simulink model "Practica_3_slm"  (R2022a)
settings: Solver=VariableStepAuto  StartTime=0.0  StopTime=10.0  RelTol=1e-3
values from neighbouring files (symbols this model uses):
  b1 = 1000    [Practica_3_codigo_sml.m]    (also in Practica_3_fx.m)
  f = 0    [Practica_3_codigo_sml.m]    (also in Practica_3_fx.m)
  k1 = 16182    [Practica_3_codigo_sml.m]    (also in Practica_3_fx.m)
  k2 = 19000    [Practica_3_codigo_sml.m]    (also in Practica_3_fx.m)
  m1 = 290    [Practica_3_codigo_sml.m]    (also in Practica_3_fx.m)
  m2 = 59    [Practica_3_codigo_sml.m]    (also in Practica_3_fx.m)
libraries: fl_lib x11, nesl_utility x4
settings Model: Creator=Peri_XP  LastModifiedBy=Peri_XP

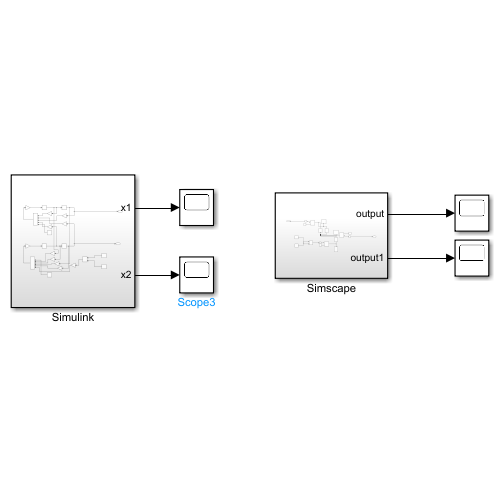
[thumbnail: Simulink's stored preview of the top-level diagram]
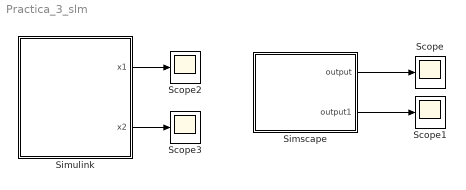
== system Practica_3_slm ==
  Scope{,1..3} (4 alike) : Scope
  Simscape : Subsystem
  Simulink : Subsystem
  wires:
  Simulink/1(x1) -> Scope2/1
  Simulink/2(x2) -> Scope3/1
  Simscape/1(output) -> Scope/1
  Simscape/2(output1) -> Scope1/1

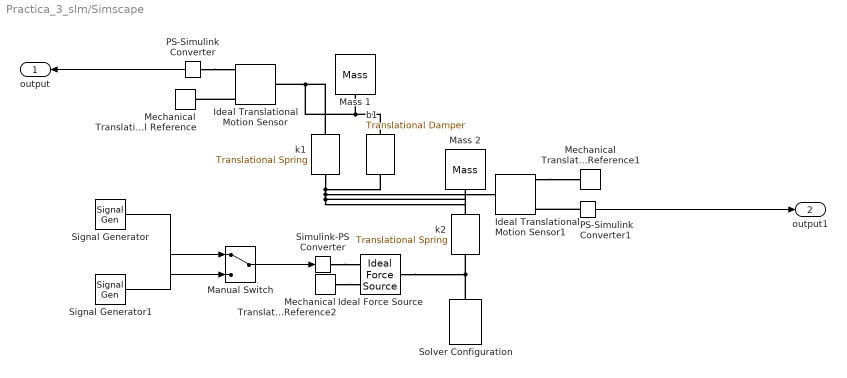
== system Practica_3_slm/Simscape ==
  Ideal Force Source : fl_lib/Mechanical/Mechanical Sources/Ideal Force Source
      settings: SourceProductBaseCode=PW,SS,VE
  Ideal Translational Motion Sensor : fl_lib/Mechanical/Mechanical Sensors/Ideal Translational Motion Sensor  offset=0 m
      settings: SourceProductBaseCode=PW,SS,VE
  Ideal Translational Motion Sensor1 : fl_lib/Mechanical/Mechanical Sensors/Ideal Translational Motion Sensor  offset=0 m
      settings: SourceProductBaseCode=PW,SS,VE
  Manual Switch : ManualSwitch
  Mass 1 : fl_lib/Mechanical/Translational Elements/Mass  mass=290 kg  num_ports=foundation.enum.numPorts2.one  v_specify=off  v_priority=High  v=0 m/s  v_nominal_specify=off  v_nominal_unit=m/s  v_nominal_value=1  f_specify=off  f_priority=None  f=0 N  f_nominal_specify=off  f_nominal_unit=N  f_nominal_value=1
      settings: SourceProductBaseCode=PW,SS,VE
  Mass 2 : fl_lib/Mechanical/Translational Elements/Mass  mass=59 kg  num_ports=foundation.enum.numPorts2.one  v_specify=off  v_priority=High  v=0 m/s  v_nominal_specify=off  v_nominal_unit=m/s  v_nominal_value=1  f_specify=off  f_priority=None  f=0 N  f_nominal_specify=off  f_nominal_unit=N  f_nominal_value=1
      settings: SourceProductBaseCode=PW,SS,VE
  Mechanical Translational Reference : fl_lib/Mechanical/Translational Elements/Mechanical Translational Reference
      settings: SourceProductBaseCode=PW,SS,VE
  Mechanical Translational Reference1 : fl_lib/Mechanical/Translational Elements/Mechanical Translational Reference
      settings: SourceProductBaseCode=PW,SS,VE
  Mechanical Translational Reference2 : fl_lib/Mechanical/Translational Elements/Mechanical Translational Reference
      settings: SourceProductBaseCode=PW,SS,VE
  PS-Simulink Converter : nesl_utility/PS-Simulink Converter  PhysicalDomain=network_engine_domain  SubClassName=ps_output  LeftPortType=input  RightPortType=output  PseudoPeriodic=off  Frequencies=[]  VectorFormat=inherit  Unit=inherit  AffineConversion=off
      settings: SourceProductBaseCode=SS,PW,VE
  PS-Simulink Converter1 : nesl_utility/PS-Simulink Converter  PhysicalDomain=network_engine_domain  SubClassName=ps_output  LeftPortType=input  RightPortType=output  PseudoPeriodic=off  Frequencies=[]  VectorFormat=inherit  Unit=inherit  AffineConversion=off
      settings: SourceProductBaseCode=SS,PW,VE
  Signal Generator : SignalGenerator  Amplitude=0.05  Frequency=0.5*pi  Units=rad/sec
  Signal Generator1 : SignalGenerator  Amplitude=0.05  Frequency=20*pi  Units=rad/sec
  Simulink-PS Converter : nesl_utility/Simulink-PS Converter  PhysicalDomain=network_engine_domain  SubClassName=ps_input  LeftPortType=input  RightPortType=output  PseudoPeriodic=off  Frequencies=[]  NoiseDistribution=none  NoiseParameters=[]  Unit=1  AffineConversion=off  FilteringAndDerivatives=provide  SimscapeFilterOrder=1  InputFilterTimeConstant=0.001  UdotUserProvided=0
      settings: SourceProductBaseCode=SS,PW,VE
  Solver Configuration : nesl_utility/Solver Configuration  PhysicalDomain=network_engine_domain  SubClassName=solver  LeftPortType=input  RightPortType=generic  Tones=[]  Harmonics=[]  SimulateNoise=off  Profile=off  UseLocalSampling=off  EnableSwitchedLinearOptims=on  FrequencyDomain=off  UseCCode=off  RelTol=0.001  AbsTol=0.001  MinStep=1e-09  ToWorkspace=off  RevertToSquareIcSolve=off  NumHomotopyIterations=100  PhasorMode=off  PhasorModeNumHarmonics=1  IndexReductionMethod=DerivativeReplacement  DoDC=off  ResidualTolerance=1e-09  UseLocalSolver=off  LocalSolverChoice=NE_BACKWARD_EULER_ADVANCER  LocalSolverSampleTime=0.001  DoFixedCost=off  MaxNonlinIter=3  MaxModeIter=2  ComputeImpulses=off  ImpulseIterations=2  LinearAlgebra=auto  LinearAlgebraNumThread=0  EquationFormulation=NE_TIME_EF  DelaysMemoryBudget=1024  AutomaticFiltering=on  FilteringTimeConstant=0.001  PartitionStorageMethod=AS_NEEDED  PartitionMemoryBudget=1024  PartitionMethod=ROBUST
      settings: SourceProductBaseCode=SS,PW,VE
  b1 : fl_lib/Mechanical/Translational Elements/Translational Damper  D=1000 N*s/m  v_specify=off  v_priority=None  v=0 m/s  v_nominal_specify=off  v_nominal_unit=m/s  v_nominal_value=1  f_specify=off  f_priority=None  f=0 N  f_nominal_specify=off  f_nominal_unit=N  f_nominal_value=1
      settings: SourceProductBaseCode=PW,SS,VE
  k1 : fl_lib/Mechanical/Translational Elements/Translational Spring  spr_rate=16182 N/m  v_specify=off  v_priority=None  v=0 m/s  v_nominal_specify=off  v_nominal_unit=m/s  v_nominal_value=1  f_specify=off  f_priority=None  f=0 N  f_nominal_specify=off  f_nominal_unit=N  f_nominal_value=1  x_specify=off  x_priority=High  x=0 m  x_nominal_specify=off  x_nominal_unit=m  x_nominal_value=1
      settings: SourceProductBaseCode=PW,SS,VE
  k2 : fl_lib/Mechanical/Translational Elements/Translational Spring  spr_rate=19000 N/m  v_specify=off  v_priority=None  v=0 m/s  v_nominal_specify=off  v_nominal_unit=m/s  v_nominal_value=1  f_specify=off  f_priority=None  f=0 N  f_nominal_specify=off  f_nominal_unit=N  f_nominal_value=1  x_specify=off  x_priority=High  x=0 m  x_nominal_specify=off  x_nominal_unit=m  x_nominal_value=1
      settings: SourceProductBaseCode=PW,SS,VE
  output : Outport
  output1 : Outport  Port=2
  wires:
  Signal Generator1/1 -> Manual Switch/1
  Manual Switch/1 -> Simulink-PS Converter/1
  Signal Generator/1 -> Manual Switch/2
  PS-Simulink Converter/1 -> output/1
  PS-Simulink Converter1/1 -> output1/1
  connections:
  k1/RConn1 -- b1/RConn1 -- Mass 1/LConn1 -- Ideal Translational Motion Sensor/LConn1
  Ideal Translational Motion Sensor1/RConn1 -- Mechanical Translational Reference1/LConn1
  k1/LConn1 -- k2/RConn1 -- Mass 2/LConn1 -- Ideal Translational Motion Sensor1/LConn1 -- b1/LConn1
  Simulink-PS Converter/RConn1 -- Ideal Force Source/RConn1
  Ideal Translational Motion Sensor/RConn1 -- Mechanical Translational Reference/LConn1
  PS-Simulink Converter/LConn1 -- Ideal Translational Motion Sensor/RConn3
  PS-Simulink Converter1/LConn1 -- Ideal Translational Motion Sensor1/RConn3
  Solver Configuration/RConn1 -- k2/LConn1 -- Ideal Force Source/LConn1
  Mechanical Translational Reference2/LConn1 -- Ideal Force Source/RConn2

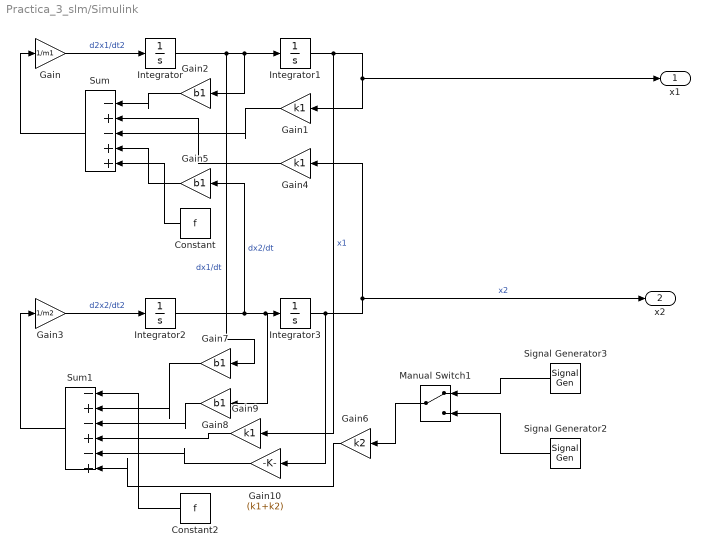
== system Practica_3_slm/Simulink ==
  Constant : Constant  Value=f
  Constant2 : Constant  Value=f
  Gain : Gain  Gain=1/m1
  Gain1 : Gain  Gain=k1
  Gain10 : Gain  Gain=(k1+k2)
  Gain{2,5,7..8} (4 alike) : Gain  Gain=b1
  Gain3 : Gain  Gain=1/m2
  Gain4 : Gain  Gain=k1
  Gain6 : Gain  Gain=k2
  Gain9 : Gain  Gain=k1
  Integrator{,1..3} (4 alike) : Integrator
  Manual Switch1 : ManualSwitch
  Signal Generator2 : SignalGenerator  Amplitude=0.05  Frequency=0.5*pi  Units=rad/sec
  Signal Generator3 : SignalGenerator  Amplitude=0.05  Frequency=20*pi  Units=rad/sec
  Sum : Sum  Inputs=|-+-++
  Sum1 : Sum  Inputs=|-+-+-+
  x1 : Outport
  x2 : Outport  Port=2
  wires:
  Integrator3/1 -> Gain10/1, x2/1, Gain4/1  "x2"
  Constant2/1 -> Sum1/1
  Gain5/1 -> Sum/4
  Integrator1/1 -> x1/1, Gain1/1, Gain9/1  "x1"
  Gain9/1 -> Sum1/4
  Integrator2/1 -> Gain5/1, Gain8/1, Integrator3/1  "dx2/dt"
  Integrator/1 -> Gain7/1, Gain2/1, Integrator1/1  "dx1/dt"
  Gain/1 -> Integrator/1  "d2x1/dt2"
  Gain4/1 -> Sum/2
  Signal Generator3/1 -> Manual Switch1/1
  Sum/1 -> Gain/1
  Gain3/1 -> Integrator2/1  "d2x2/dt2"
  Signal Generator2/1 -> Manual Switch1/2
  Sum1/1 -> Gain3/1
  Gain1/1 -> Sum/3
  Gain7/1 -> Sum1/2
  Gain8/1 -> Sum1/3
  Manual Switch1/1 -> Gain6/1
  Gain2/1 -> Sum/1
  Gain6/1 -> Sum1/6
  Gain10/1 -> Sum1/5
  Constant/1 -> Sum/5
